simulink model "test2"  (R2017b)
settings: Solver=VariableStepAuto  StartTime=0.0  StopTime=10.0  RelTol=1e-3
settings Model: Creator=flosch  LastModifiedBy=flosch

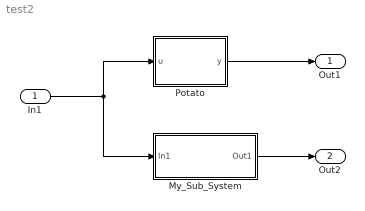
== system test2 ==
  In1 : Inport
  My_Sub_System : Subsystem
  Potato : MATLAB Function  TreatAsAtomicUnit=on
  Out1 : Outport
  Out2 : Outport  Port=2
  wires:
  In1/1 -> My_Sub_System/1(In1), Potato/1(u)
  Potato/1(y) -> Out1/1
  My_Sub_System/1(Out1) -> Out2/1

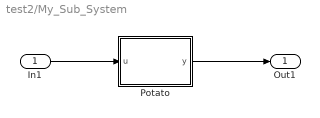
== system test2/My_Sub_System ==
  In1 : Inport
  Potato : MATLAB Function  TreatAsAtomicUnit=on
  Out1 : Outport
  wires:
  In1/1 -> Potato/1(u)
  Potato/1(y) -> Out1/1

== matlab function test2/My_Sub_System/Potato ==
  data: u input; y output
function y = fcn(u)
% This is in the subsystem
y = u;

== matlab function test2/Potato ==
  data: u input; y output
function y = fcn(u)
% This is in test2
y = u;
